simulink model "PIDsimu"  (R2020b)
settings: Solver=VariableStepAuto  StartTime=0.0  StopTime=30  RelTol=1e-3
undefined symbols (not defined in the file or in its folder): km, Kp, kt, kTP, kTV, Kv, Ra, Tm, Tv
libraries: simulink x1
settings Model: Creator=My Computer  LastModifiedBy=My Computer

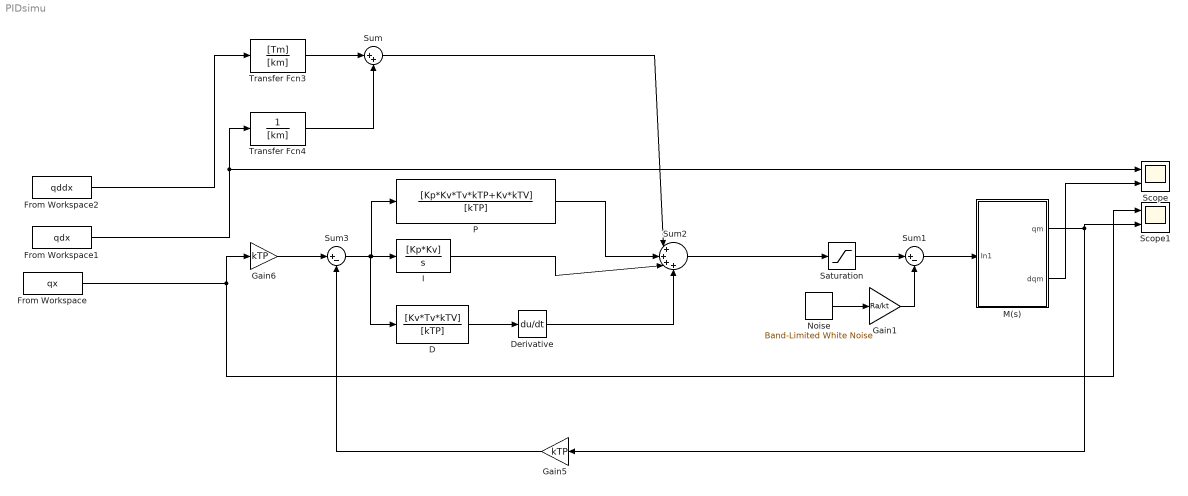
== system PIDsimu ==
  D : TransferFcn  Numerator=[Kv*Tv*kTV]  Denominator=[kTP]
  Derivative : Derivative
  From Workspace : FromWorkspace  VariableName=qx
  From Workspace1 : FromWorkspace  VariableName=qdx
  From Workspace2 : FromWorkspace  VariableName=qddx
  Gain1 : Gain  Gain=Ra/kt
  Gain5 : Gain  Gain=kTP
  Gain6 : Gain  Gain=kTP
  I : TransferFcn  Numerator=[Kp*Kv]  Denominator=[1 0]
  M(s) : Subsystem
  Noise : simulink/Sources/Band-Limited White Noise  Cov=[0.1]  Ts=0.1  seed=[23341]
  P : TransferFcn  Numerator=[Kp*Kv*Tv*kTP+Kv*kTV]  Denominator=[kTP]
  Saturation : Saturate  UpperLimit=1000  LowerLimit=-1000
  Scope : Scope  NumInputPorts=2
  Scope1 : Scope  NumInputPorts=2
  Sum : Sum  Inputs=|++
  Sum1 : Sum  Inputs=|+-
  Sum2 : Sum  Inputs=|++++
  Sum3 : Sum  Inputs=|+-
  Transfer Fcn3 : TransferFcn  Numerator=[Tm]  Denominator=[km]
  Transfer Fcn4 : TransferFcn  Denominator=[km]
  wires:
  P/1 -> Sum2/2
  Noise/1 -> Gain1/1
  Derivative/1 -> Sum2/4
  I/1 -> Sum2/3
  Gain6/1 -> Sum3/1
  From Workspace1/1 -> Transfer Fcn4/1, Scope/1
  D/1 -> Derivative/1
  Sum2/1 -> Saturation/1
  Transfer Fcn3/1 -> Sum/1
  Sum/1 -> Sum2/1
  Gain1/1 -> Sum1/2
  From Workspace/1 -> Scope1/1, Gain6/1
  Sum1/1 -> M(s)/1(In1)
  Transfer Fcn4/1 -> Sum/2
  Sum3/1 -> D/1, I/1, P/1
  From Workspace2/1 -> Transfer Fcn3/1
  Saturation/1 -> Sum1/1
  M(s)/1(qm) -> Scope1/2, Gain5/1
  Gain5/1 -> Sum3/2
  M(s)/2(dqm) -> Scope/2

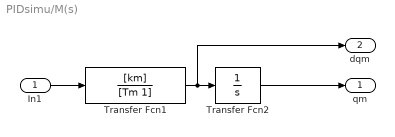
== system PIDsimu/M(s) ==
  In1 : Inport
  Transfer Fcn1 : TransferFcn  Numerator=[km]  Denominator=[Tm 1]
  Transfer Fcn2 : TransferFcn  Denominator=[1 0]
  qm : Outport
  dqm : Outport  Port=2
  wires:
  Transfer Fcn1/1 -> dqm/1, Transfer Fcn2/1
  In1/1 -> Transfer Fcn1/1
  Transfer Fcn2/1 -> qm/1
